simulink model "bus_creator_and_selector"  (R2018b)
settings: Solver=FixedStepDiscrete  StartTime=0.0  StopTime=10.0  RelTol=1e-3
libraries: simulink x3
settings Model: Creator=marwan  LastModifiedBy=marwan

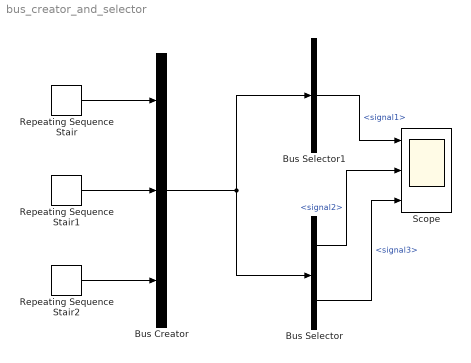
== system bus_creator_and_selector ==
  Bus Creator : BusCreator  Inputs=3
  Bus Selector : BusSelector  OutputSignals=signal2,signal3
  Bus Selector1 : BusSelector  OutputSignals=signal1
  Repeating Sequence Stair : simulink/Sources/Repeating Sequence Stair  OutValues=[1 2 3 4 5]  tsamp=-1  OutMin=[]  OutMax=[]  OutDataTypeStr=double  OutputDataTypeScalingMode=double  OutDataType=fixdt(0,8)  ConRadixGroup=Best Precision: Vector-wise  OutScaling=2^-12
  Repeating Sequence Stair1 : simulink/Sources/Repeating Sequence Stair  OutValues=[6 7 8 9 10]  tsamp=-1  OutMin=[]  OutMax=[]  OutDataTypeStr=double  OutputDataTypeScalingMode=double  OutDataType=fixdt(0,8)  ConRadixGroup=Best Precision: Vector-wise  OutScaling=2^-12
  Repeating Sequence Stair2 : simulink/Sources/Repeating Sequence Stair  OutValues=[11 12 13 14 15]  tsamp=-1  OutMin=[]  OutMax=[]  OutDataTypeStr=double  OutputDataTypeScalingMode=double  OutDataType=fixdt(0,8)  ConRadixGroup=Best Precision: Vector-wise  OutScaling=2^-12
  Scope : Scope  NumInputPorts=3
  wires:
  Repeating Sequence Stair/1 -> Bus Creator/1
  Repeating Sequence Stair1/1 -> Bus Creator/2
  Repeating Sequence Stair2/1 -> Bus Creator/3
  Bus Creator/1 -> Bus Selector1/1, Bus Selector/1
  Bus Selector1/1 -> Scope/1  "<signal1>"
  Bus Selector/1 -> Scope/2  "<signal2>"
  Bus Selector/2 -> Scope/3  "<signal3>"
